simulink model "Homework_3"  (R2023b)
settings: Solver=FixedStepDiscrete  StartTime=0.0  StopTime=1  FixedStep=0.002  RelTol=1e-3  EnableMultiTasking=on
values from neighbouring files (symbols this model uses):
  a = [-1 ; 1 ; -sqrt(3)]    [Inputs_to_simulink.m]
  alpha = 104.47    [Inputs_to_simulink.m]
  Beta = [B_0 ; B_1 ; B_2 ; B_3]    [Inputs_to_simulink.m]
  phi = 90    [Inputs_to_simulink.m]
  psi = 90    [Inputs_to_simulink.m]
  theta = 45    [Inputs_to_simulink.m]
undefined symbols (not defined in the file or in its folder): R
settings Model: ExtModeTrigDuration=10000  Creator=jtmil  LastModifiedBy=jtmil
settings SolverCC: AlgebraicLoopSolver=TrustRegion  PositivePriorityOrder=on
settings DataIOCC: ReturnWorkspaceOutputs=off
settings OptimizationCC: LifeSpan=inf
settings DebuggingCC: UnconnectedInputMsg=warning  UnconnectedOutputMsg=warning  UnconnectedLineMsg=warning  ArithmeticOperatorsInVariantConditions=warning
settings ModelReferenceCC: EnableRefExpFcnMdlSchedulingChecks=on
settings SFSimCC: SimUseLocalCustomCode=off  CustomCodeUndefinedFunction=UseInterfaceOnly
settings RTWCC: Description=QUARC Win64 Target  SystemTargetFile=quarc_win64.tlc  TemplateMakefile=quarc_default_tmf  RTWUseLocalCustomCode=off
settings CodeAppCC: StateflowObjectComments=on
settings STFCustomTargetCC: TargetPreCompLibLocation=C:\PROGRA~3\QUARC\lib\2016a\win64\release  ConcurrentExecutionCompliant=on  GRTInterface=on  SystemTargetFile=quarc_win64.tlc
settings GRTTargetCC: TargetPreCompLibLocation=C:\PROGRA~3\QUARC\lib\2016a\win64\release  ParMdlRefBuildCompliant=off  CompOptLevelCompliant=off  CombineOutputUpdateFcns=off  MatFileLogging=off  CPPClassGenCompliant=off  GRTInterface=on  UseToolchainInfoCompliant=off  ExtMode=on  ExtModeMexFile=quarc_comm
settings ConfigComp: CovMetricSettings=dswe

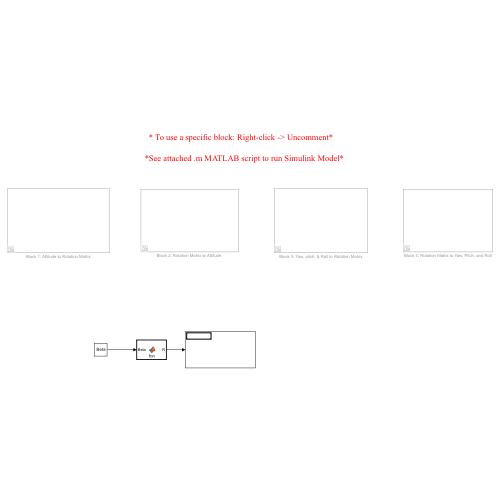
[thumbnail: Simulink's stored preview of the top-level diagram]
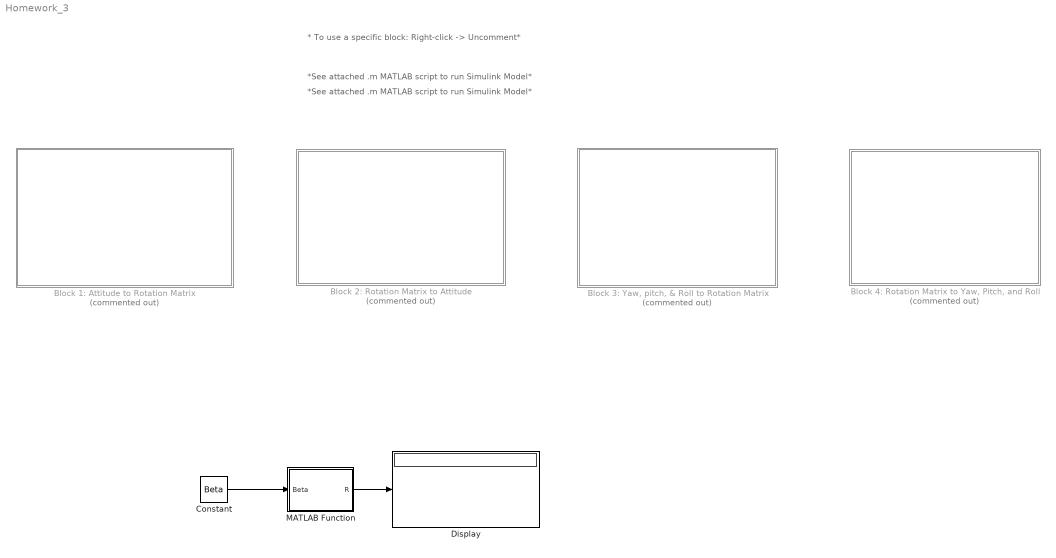
== system Homework_3 ==
  note: *See attached .m MATLAB script to run Simulink Model*
  note: * To use a specific block: Right-click -> Uncomment*
  note: *See attached .m MATLAB script to run Simulink Model*
  Block 1: Attitude to Rotation Matrix : Subsystem  Commented=on
  "Block 2: Rotation Matrix to Attitude " : Subsystem  Commented=on
  "Block 3: Yaw, pitch, & Roll to Rotation Matrix" : Subsystem  Commented=on
  "Block 4: Rotation Matrix to Yaw, Pitch, and Roll" : Subsystem  Commented=on
  Constant : Constant  Value=Beta
  Display : Display
  MATLAB Function : MATLAB Function  TreatAsAtomicUnit=on
  wires:
  Constant/1 -> MATLAB Function/1(Beta)
  MATLAB Function/1(R) -> Display/1

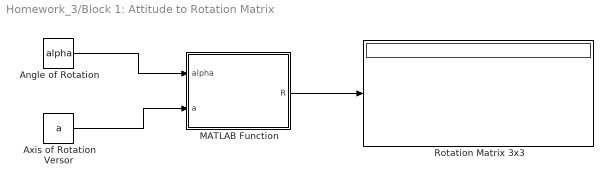
== system Homework_3/Block 1: Attitude to Rotation Matrix ==
  Angle of Rotation : Constant  Value=alpha
  Axis of Rotation Versor : Constant  Value=a
  MATLAB Function : MATLAB Function  TreatAsAtomicUnit=on
  Rotation Matrix 3x3 : Display
  wires:
  MATLAB Function/1(R) -> Rotation Matrix 3x3/1
  Axis of Rotation Versor/1 -> MATLAB Function/2(a)
  Angle of Rotation/1 -> MATLAB Function/1(alpha)

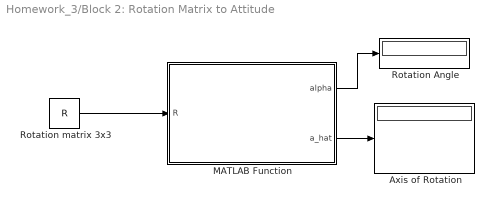
== system Homework_3/Block 2: Rotation Matrix to Attitude  ==
  Axis of Rotation : Display
  MATLAB Function : MATLAB Function  TreatAsAtomicUnit=on
  Rotation Angle : Display
  Rotation matrix 3x3 : Constant  Value=R
  wires:
  Rotation matrix 3x3/1 -> MATLAB Function/1(R)
  MATLAB Function/1(alpha) -> Rotation Angle/1
  MATLAB Function/2(a_hat) -> Axis of Rotation/1

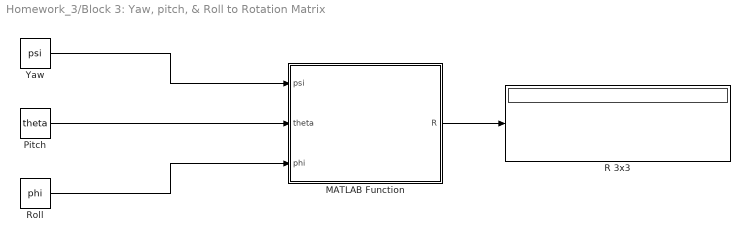
== system Homework_3/Block 3: Yaw, pitch, & Roll to Rotation Matrix ==
  MATLAB Function : MATLAB Function  TreatAsAtomicUnit=on
  Pitch : Constant  Value=theta
  R 3x3 : Display
  Roll : Constant  Value=phi
  Yaw : Constant  Value=psi
  wires:
  Yaw/1 -> MATLAB Function/1(psi)
  Pitch/1 -> MATLAB Function/2(theta)
  Roll/1 -> MATLAB Function/3(phi)
  MATLAB Function/1(R) -> R 3x3/1

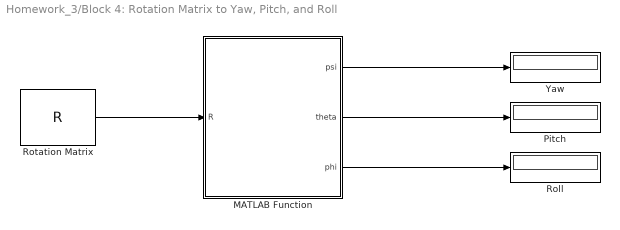
== system Homework_3/Block 4: Rotation Matrix to Yaw, Pitch, and Roll ==
  MATLAB Function : MATLAB Function  TreatAsAtomicUnit=on
  Pitch : Display
  Roll : Display
  Rotation Matrix : Constant  Value=R
  Yaw : Display
  wires:
  Rotation Matrix/1 -> MATLAB Function/1(R)
  MATLAB Function/1(psi) -> Yaw/1
  MATLAB Function/2(theta) -> Pitch/1
  MATLAB Function/3(phi) -> Roll/1

== matlab function Homework_3/Block 1: Attitude to Rotation Matrix/MATLAB Function ==
  data: alpha input; R output; a input
function R  = fcn(alpha, a)

a_hat = a/norm(a);               % Normalize vector a
a_hat_transpose = a_hat';        % Transpose Vector a
a_skew_symmetric = [0 -a(3) a(2); a(3) 0 -a(1); -a(2) a(1) 0]; % Skew Symmetric Matrix of a
I = eye(3);                       % Identity Matrix

R = cosd(alpha)*I + (1-cosd(alpha))*(a_hat*a_hat_transpose) - sind(alpha)*a_skew_symmetric; % Euler's Formula



end

== matlab function Homework_3/Block 2: Rotation Matrix to Attitude /MATLAB Function ==
  data: R input; alpha output; a_hat output
function [alpha, a_hat] = fcn(R)

% Initialize alpha and a_hat
alpha = acosd((1/2)*(R(1,1) + R(2,2) + R(3,3) - 1));


a_hat = [1; 0; 0]; 

if alpha == 0  
    a_hat = [1; 0; 0];
elseif alpha == 180
    if R(1,1) ~= -1
        a_hat_x = abs(sqrt((R(1,1) + 1) / 2));
        a_hat = [a_hat_x; R(1,2) / (2 * a_hat_x); R(1,3) / (2 * a_hat_x)];
    elseif R(2,2) ~= -1
        a_hat_y = abs(sqrt((R(2,2) + 1) / 2));
        a_hat = [R(2,1) / (2 * a_hat_y); a_hat_y; R(2,3) / (2 * a_hat_y)];
    elseif R(3,3) ~= -1
        a_hat_z = abs(sqrt((R(3,3) + 1) / 2));
        a_hat = [R(3,1) / (2 * a_hat_z); R(3,2) / (2 * a_hat_z); a_hat_z];
    end
elseif alpha > 0 && alpha < 180
    a_hat = (1 / (2 * sind(alpha))) * [R(2,3) - R(3,2); R(3,1) - R(1,3); R(1,2) - R(2,1)];
end

end

== matlab function Homework_3/Block 3: Yaw, pitch, & Roll to Rotation Matrix/MATLAB Function ==
  data: psi input; R output; theta input; phi input
function R  = fcn(psi,theta, phi)

R1 = [ 1 0 0  ; 0 cosd(phi) sind(phi) ; 0 -sind(phi) cosd(phi)];
R2 = [cosd(theta) 0 -sind(theta); 0 1 0; sind(theta) 0 cosd(theta)];
R3 = [ cosd(psi) sind(psi) 0 ; -sind(psi) cosd(psi) 0 ; 0 0 1];

R = R1*R2*R3

end

== matlab function Homework_3/Block 4: Rotation Matrix to Yaw, Pitch, and Roll/MATLAB Function ==
  data: R input; psi output; theta output; phi output
function [psi,theta,phi] = fcn(R)

phi = atan2d(R(1,2) , R(1,1)) % Yaw
theta = asind(-R(1,3))        % Pitch
psi = atan2d(R(2,3),R(3,3))   % Roll

end

== matlab function Homework_3/MATLAB Function ==
  data: Beta input; R output
function R  = fcn(Beta)
    
R= [Beta(1)^2 + Beta(2)^2 - Beta(3)^2 - Beta(4)^2 , 2*Beta(2)*Beta(3) + 2*Beta(1)*Beta(4) , 2*Beta(2)*Beta(4)-2*Beta(1)*Beta(3);
     2*Beta(2)*Beta(3) - 2*Beta(1)*Beta(4) , Beta(1)^2 - Beta(2)^2 + Beta(3)^2 -beta(4)^2 ; 2*Beta(3)*Beta(4) + 2*Beta(1)*Beta(2);
     2*Beta(2)*Beta(4) + 2*Beta(1)*Beta(3) , 2*Beta(3)*Beta(4) - 2*Beta(1)*Beta(2) , Beta(1)^2 - Beta(2)^2 - Beta(3)^2 + Beta(3)^2];


end
